simulink model "system_mpc"  (Simulink 7.9)
settings: Solver=ode45  StartTime=0.0  StopTime=10.0  RelTol=1e-3
undefined symbols (not defined in the file or in its folder): tower
libraries: mpclib x1
settings Model: Creator=matias  LastModifiedBy=matias

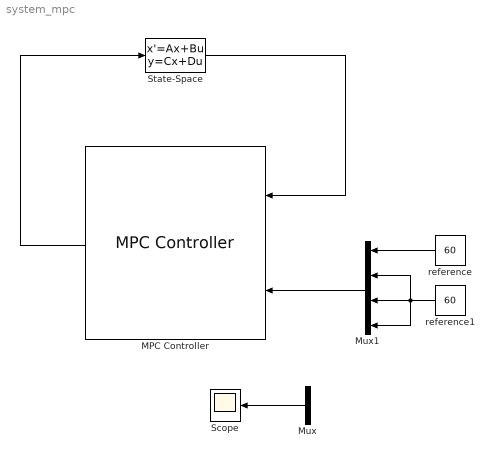
== system system_mpc ==
  MPC Controller : mpclib/MPC Controller  mpcobj=MPC1  x0=[]  md_inport=off  mv_inport=off  lims_inport=off  switch_inport=off  ywt_inport=off  duwt_inport=off  rhoeps_inport=off  cost_outport=off  return_sequence=off  return_qpstatus=off  is_multiple=0  enable_value=0  n_mv=1  n_mo=2  n_md=0  n_ts=0.01  is_designfromscratch=0  ref_from_ws=off  ref_signal_name=[]  ref_preview=on  md_from_ws=off  md_signal_name=[]  md_preview=on  from_project=off  project_file=MPCtask.mat
  Mux : Mux  Inputs=2
  Mux1 : Mux
  Scope : Scope
  State-Space : StateSpace  A=tower.A  B=tower.B  C=tower.C  D=tower.D  X0=tower.x0
  reference : Constant  Value=60
  reference1 : Constant  Value=60
  wires:
  State-Space/1 -> MPC Controller/1
  MPC Controller/1 -> State-Space/1
  Mux/1 -> Scope/1
  reference/1 -> Mux1/1
  reference1/1 -> Mux1/2, Mux1/3, Mux1/4
  Mux1/1 -> MPC Controller/2
